simulink model "Fuck"  (R2015b)
settings: Solver=FixedStepAuto  StartTime=0.0  StopTime=10  RelTol=1e-3
settings Model: Creator=bryanguner  LastModifiedBy=bryanguner

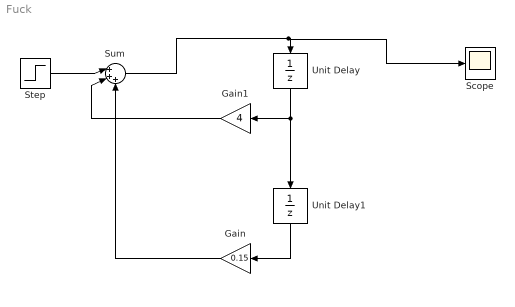
== system Fuck ==
  Gain : Gain  Gain=0.15
  Gain1 : Gain  Gain=4
  Scope : Scope
  Step : Step  SampleTime=0
  Sum : Sum  Inputs=|+++
  Unit Delay : UnitDelay  SampleTime=-1
  Unit Delay1 : UnitDelay  SampleTime=-1
  wires:
  Step/1 -> Sum/1
  Sum/1 -> Scope/1, Unit Delay/1
  Unit Delay/1 -> Unit Delay1/1, Gain1/1
  Gain1/1 -> Sum/2
  Unit Delay1/1 -> Gain/1
  Gain/1 -> Sum/3
